simulink model "sim_tcyb_2024_pos_ctrl"  (R2020a)
settings: Solver=ode4  StartTime=0.0  StopTime=30.0  FixedStep=0.01  RelTol=1e-3
values from neighbouring files (symbols this model uses):
  alfa_theta = 20    [init_tcyb_2024_pos_ctrl.m]
  alfa_theta_obs = 100    [init_tcyb_2024_pos_ctrl.m]
  c1_diff_sigma_bar_v = diag([25; 30; 20])    [init_tcyb_2024_pos_ctrl.m]
  c1v = diag([5.8; 6.5; 6.5])    [init_tcyb_2024_pos_ctrl.m]
  c2_diff_sigma_bar_v = diag([50; 50; 10])    [init_tcyb_2024_pos_ctrl.m]
  c2v = diag([5.8; 6.5; 6.5])    [init_tcyb_2024_pos_ctrl.m]
  c3_diff_sigma_bar_v = diag([15; 15; 10])    [init_tcyb_2024_pos_ctrl.m]
  c3v = diag([4.8; 6.4; 6.0])    [init_tcyb_2024_pos_ctrl.m]
  c_psi_p = [0.05; 0.05; 0.05]    [init_tcyb_2024_pos_ctrl.m]
  delta_p_i_0 = zeros(3, NF)    [init_tcyb_2024_pos_ctrl.m]
  delta_v_i_0 = zeros(3, NF)    [init_tcyb_2024_pos_ctrl.m]
  dp_aa_t = 0.2 * ones(3, 5) + ( 1.0 - 0.2 ) * rand(3, 5)    [init_tcyb_2024_pos_ctrl.m]
  dp_ff_t = [ 0.4 * ones(1, 5) + ( 1.0 - 0.4 ) * rand(1, 5);                      0.4 * ones(1, 5) + ( 1.0 - 0.4 ) * rand(1, 5);                      0.2 * ones(1, 5) + ( 0.6 - 0.2 ) * rand(1, 5) ]    [init_tcyb_2024_pos_ctrl.m]
  dp_phi_t = ( - pi / 2 ) * ones(3, 5) + ( pi / 2 - ( - pi / 2 ) ) * rand(3, 5)    [init_tcyb_2024_pos_ctrl.m]
  etai_0 = zeros(3,5)    [init_tcyb_2024_pos_ctrl.m]
  kai_1_t = 0.02    [init_tcyb_2024_pos_ctrl.m]
  kai_3_t = 0.1    [init_tcyb_2024_pos_ctrl.m]
  ksii_0 = zeros(3,5)    [init_tcyb_2024_pos_ctrl.m]
  l1v = diag([20; 20; 20])    [init_tcyb_2024_pos_ctrl.m]
  l2v = diag([30; 30; 30])    [init_tcyb_2024_pos_ctrl.m]
  Lamd_diff_sigma_bar_v = 0.5    [init_tcyb_2024_pos_ctrl.m]
  mass_i = zeros(1,NF)    [init_tcyb_2024_pos_ctrl.m]
  Mii = diag([1;0;0;0;1])    [init_tcyb_2024_pos_ctrl.m]
  pos0 = zeros(3, 1)    [init_tcyb_2024_pos_ctrl.m]
  PZ0 = P0(3)    [init_tcyb_2024_pos_ctrl.m]
  PZ1 = 10    [init_tcyb_2024_pos_ctrl.m]
  Qci_init = repmat([1;0;0;0],1,NF)    [init_tcyb_2024_pos_ctrl.m]
  R0 = 4    [init_tcyb_2024_pos_ctrl.m]
  R1 = 8    [init_tcyb_2024_pos_ctrl.m]
  rho_p = [0.1; 0.1; 0.1]    [init_tcyb_2024_pos_ctrl.m]
  Rx2 = 10    [init_tcyb_2024_pos_ctrl.m]
  Ry2 = 6    [init_tcyb_2024_pos_ctrl.m]
  Rz2 = 4    [init_tcyb_2024_pos_ctrl.m]
  T0 = 0    [init_tcyb_2024_pos_ctrl.m]
  T1 = tseq1    (= 10)    [init_tcyb_2024_pos_ctrl.m]
  T12 = tseq1 + tseq12    (= 20)    [init_tcyb_2024_pos_ctrl.m]
  T2 = tseq1 + tseq12 + tseq2    (= 30)    [init_tcyb_2024_pos_ctrl.m]
  tau_p = 5    [init_tcyb_2024_pos_ctrl.m]
  theta0 = ( 2 / 5 ) * pi    (= 1.25663706144)    [init_tcyb_2024_pos_ctrl.m]
  vel0 = zeros(3, 1)    [init_tcyb_2024_pos_ctrl.m]
  Wij = [0,0,1,0,0;              0,0,1,1,0;              1,0,0,0,1;              0,1,1,0,0;              0,0,1,0,0]    [init_tcyb_2024_pos_ctrl.m]
  X1 = 8    [init_tcyb_2024_pos_ctrl.m]
  X2 = 2    [init_tcyb_2024_pos_ctrl.m]
  X3 = 3    [init_tcyb_2024_pos_ctrl.m]
  Y1 = 10    [init_tcyb_2024_pos_ctrl.m]
  Y2 = 2    [init_tcyb_2024_pos_ctrl.m]
  Y3 = 4    [init_tcyb_2024_pos_ctrl.m]
  Z1 = 4    [init_tcyb_2024_pos_ctrl.m]
  Z2 = -6    [init_tcyb_2024_pos_ctrl.m]
  Z3 = 2    [init_tcyb_2024_pos_ctrl.m]
  zeta_diff_sigma_bar_v = 0.08    [init_tcyb_2024_pos_ctrl.m]
undefined symbols (not defined in the file or in its folder): cal_frac_squ, p_alfav1, p_alfav2, p_gamma1_pos, p_gamma1_vel, p_gamma2_pos, p_gamma2_vel, q_alfav1, q_alfav2, q_gamma1_pos, q_gamma1_vel, q_gamma2_pos, q_gamma2_vel
(part 4 of 4)

== matlab function sim_tcyb_2024_pos_ctrl/trans to column51 ==
  data: x input; y output
function y = fcn(x)
y = x(:);

== matlab function sim_tcyb_2024_pos_ctrl/eta_p_hat adaptive law agent 4 ==
  data: tau_p input; tsim input; d_eta_p_hat_4 output; err_lump_vec input; eta_p_hat_vec input
function d_eta_p_hat_4 = fcn(tau_p, tsim, err_lump_vec, eta_p_hat_vec)
%%%% 计算自适应律
iiuav = 4;
d_eta_p_hat_4 = tau_p * norm(err_lump_vec(:,iiuav), 2) ...
                                - ( 0.1 * exp(-tsim) ) * tau_p .* eta_p_hat_vec(iiuav);

== matlab function sim_tcyb_2024_pos_ctrl/trans to column52 ==
  data: x input; y output
function y = fcn(x)
y = x(:);

== matlab function sim_tcyb_2024_pos_ctrl/trans to column53 ==
  data: x input; y output
function y = fcn(x)
y = x(:);

== matlab function sim_tcyb_2024_pos_ctrl/trans to column54 ==
  data: x input; y output
function y = fcn(x)
y = x(:);

== matlab function sim_tcyb_2024_pos_ctrl/trans to column55 ==
  data: x input; y output
function y = fcn(x)
y = x(:);

== matlab function sim_tcyb_2024_pos_ctrl/trans to column56 ==
  data: x input; y output
function y = fcn(x)
y = x(:);

== matlab function sim_tcyb_2024_pos_ctrl/trans to column57 ==
  data: x input; y output
function y = fcn(x)
y = x(:);

== matlab function sim_tcyb_2024_pos_ctrl/trans to column58 ==
  data: x input; y output
function y = fcn(x)
y = x(:);

== matlab function sim_tcyb_2024_pos_ctrl/trans to column59 ==
  data: x input; y output
function y = fcn(x)
y = x(:);

== matlab function sim_tcyb_2024_pos_ctrl/trans to column60 ==
  data: x input; y output
function y = fcn(x)
y = x(:);

== matlab function sim_tcyb_2024_pos_ctrl/eta_p_hat adaptive law agent 5 ==
  data: tau_p input; tsim input; d_eta_p_hat_5 output; err_lump_vec input; eta_p_hat_vec input
function d_eta_p_hat_5 = fcn(tau_p, tsim, err_lump_vec, eta_p_hat_vec)
%%%% 计算自适应律
iiuav = 5;
d_eta_p_hat_5 = tau_p * norm(err_lump_vec(:,iiuav), 2) ...
                                - ( 0.1 * exp(-tsim) ) * tau_p .* eta_p_hat_vec(iiuav);

== matlab function sim_tcyb_2024_pos_ctrl/combine eta_p_hat adaptive ==
  data: eta_p_hat_1 input; eta_p_hat_vec output; eta_p_hat_2 input; eta_p_hat_3 input; eta_p_hat_4 input; eta_p_hat_5 input
function eta_p_hat_vec = fcn(eta_p_hat_1, eta_p_hat_2, eta_p_hat_3, eta_p_hat_4, eta_p_hat_5)
%%%% 合并领导者位置观测器输出结果
eta_p_hat_vec = [eta_p_hat_1, eta_p_hat_2, eta_p_hat_3, eta_p_hat_4, eta_p_hat_5];

== matlab function sim_tcyb_2024_pos_ctrl/cal auxiliary error Gi agent 1 ==
  data: tsim input; Gi_1 output; err_lump_vec input; eta_p_hat_vec input
function Gi_1 = fcn(tsim, err_lump_vec, eta_p_hat_vec)
%%%% 计算自适应律
iiuav = 1;
Gi_1 = ( ( eta_p_hat_vec(iiuav) ^ 2 ) / ...
                ( norm(err_lump_vec(:,iiuav), 2) * eta_p_hat_vec(iiuav) + 0.1 * exp(-tsim) ) ) ...
                * err_lump_vec(:,iiuav);

== matlab function sim_tcyb_2024_pos_ctrl/cal position and velocity signal tracking errors ==
  data: ksi_i_vec input; err_ksi_vec output; ksi_d_est_vec input; eta_i_vec input; eta_d_est_vec input; err_eta_vec output
function [err_ksi_vec, err_eta_vec] = fcn(ksi_i_vec, ksi_d_est_vec, eta_i_vec, eta_d_est_vec)
%%%% 计算编队跟踪误差
err_ksi_vec = zeros(3,5);
err_eta_vec = zeros(3,5);
for iiuav = 1:5
    err_ksi_vec(:,iiuav) = ksi_i_vec(:,iiuav) - ksi_d_est_vec(:,iiuav);
    err_eta_vec(:,iiuav) = eta_i_vec(:,iiuav) - eta_d_est_vec(:,iiuav);
end

== matlab function sim_tcyb_2024_pos_ctrl/cal auxiliary error Gi agent 2 ==
  data: tsim input; Gi_2 output; err_lump_vec input; eta_p_hat_vec input
function Gi_2 = fcn(tsim, err_lump_vec, eta_p_hat_vec)
%%%% 计算自适应律
iiuav = 2;
Gi_2 = ( ( eta_p_hat_vec(iiuav) ^ 2 ) / ...
                ( norm(err_lump_vec(:,iiuav), 2) * eta_p_hat_vec(iiuav) + 0.1 * exp(-tsim) ) ) ...
                * err_lump_vec(:,iiuav);

== matlab function sim_tcyb_2024_pos_ctrl/cal auxiliary error Gi agent 3 ==
  data: tsim input; Gi_3 output; err_lump_vec input; eta_p_hat_vec input
function Gi_3 = fcn(tsim, err_lump_vec, eta_p_hat_vec)
%%%% 计算自适应律
iiuav = 3;
Gi_3 = ( ( eta_p_hat_vec(iiuav) ^ 2 ) / ...
                ( norm(err_lump_vec(:,iiuav), 2) * eta_p_hat_vec(iiuav) + 0.1 * exp(-tsim) ) ) ...
                * err_lump_vec(:,iiuav);

== matlab function sim_tcyb_2024_pos_ctrl/cal auxiliary error Gi agent 4 ==
  data: tsim input; Gi_4 output; err_lump_vec input; eta_p_hat_vec input
function Gi_4 = fcn(tsim, err_lump_vec, eta_p_hat_vec)
%%%% 计算自适应律
iiuav = 4;
Gi_4 = ( ( eta_p_hat_vec(iiuav) ^ 2 ) / ...
                ( norm(err_lump_vec(:,iiuav), 2) * eta_p_hat_vec(iiuav) + 0.1 * exp(-tsim) ) ) ...
                * err_lump_vec(:,iiuav);

== matlab function sim_tcyb_2024_pos_ctrl/cal auxiliary error Gi agent 5 ==
  data: tsim input; Gi_5 output; err_lump_vec input; eta_p_hat_vec input
function Gi_5 = fcn(tsim, err_lump_vec, eta_p_hat_vec)
%%%% 计算自适应律
iiuav = 5;
Gi_5 = ( ( eta_p_hat_vec(iiuav) ^ 2 ) / ...
                ( norm(err_lump_vec(:,iiuav), 2) * eta_p_hat_vec(iiuav) + 0.1 * exp(-tsim) ) ) ...
                * err_lump_vec(:,iiuav);

== matlab function sim_tcyb_2024_pos_ctrl/combine Gi ==
  data: Gi_1 input; Gi_vec output; Gi_2 input; Gi_3 input; Gi_4 input; Gi_5 input
function Gi_vec = fcn(Gi_1, Gi_2, Gi_3, Gi_4, Gi_5)
%%%% 合并领导者位置观测器输出结果
Gi_vec = [Gi_1(:), Gi_2(:), Gi_3(:), Gi_4(:), Gi_5(:)];

== matlab function sim_tcyb_2024_pos_ctrl/cal formation tracking Gi error ==
  data: wi0 input; err_Gi_form_vec output; wij input; Gi_vec input
function err_Gi_form_vec = fcn(wi0, wij, Gi_vec)
%%%% 计算编队跟踪误差
err_Gi_form_vec = zeros(3,5);
for iiuav = 1:5
    err_Gi_form_vec(:,iiuav) = wi0(iiuav, iiuav) * Gi_vec(:,iiuav);
    for jjuav = 1:5
        err_Gi_form_vec(:,iiuav) = err_Gi_form_vec(:,iiuav) ...
                                                        + wij(iiuav, jjuav) * (Gi_vec(:,iiuav) - Gi_vec(:,jjuav));
    end
end

== matlab function sim_tcyb_2024_pos_ctrl/cal ui agent 2 ==
  data: c_psi_p input; d_delta_eta_vec input; ui_2 output; err_Gi_form_vec input; eps_p_hat_vec input; err_lump_vec input; dp_hat_vec input
function ui_2 = fcn(c_psi_p, d_delta_eta_vec, err_Gi_form_vec, eps_p_hat_vec, err_lump_vec, dp_hat_vec)
%%%% 计算控制输入ui
iiuav = 2;
g0 = 9.80663;
e3 = [0;0;1];
ui_2 = g0 * e3 + d_delta_eta_vec(:,iiuav) - c_psi_p(:) .* err_Gi_form_vec(:,iiuav) ...
            - eps_p_hat_vec(iiuav) * err_lump_vec(:,iiuav) - dp_hat_vec(:,iiuav);

== matlab function sim_tcyb_2024_pos_ctrl/cal ui agent 3 ==
  data: c_psi_p input; d_delta_eta_vec input; ui_3 output; err_Gi_form_vec input; eps_p_hat_vec input; err_lump_vec input; dp_hat_vec input
function ui_3 = fcn(c_psi_p, d_delta_eta_vec, err_Gi_form_vec, eps_p_hat_vec, err_lump_vec, dp_hat_vec)
%%%% 计算控制输入ui
iiuav = 3;
g0 = 9.80663;
e3 = [0;0;1];
ui_3 = g0 * e3 + d_delta_eta_vec(:,iiuav) - c_psi_p(:) .* err_Gi_form_vec(:,iiuav) ...
            - eps_p_hat_vec(iiuav) * err_lump_vec(:,iiuav) - dp_hat_vec(:,iiuav);

== matlab function sim_tcyb_2024_pos_ctrl/cal ui agent 4 ==
  data: c_psi_p input; d_delta_eta_vec input; ui_4 output; err_Gi_form_vec input; eps_p_hat_vec input; err_lump_vec input; dp_hat_vec input
function ui_4 = fcn(c_psi_p, d_delta_eta_vec, err_Gi_form_vec, eps_p_hat_vec, err_lump_vec, dp_hat_vec)
%%%% 计算控制输入ui
iiuav = 4;
g0 = 9.80663;
e3 = [0;0;1];
ui_4 = g0 * e3 + d_delta_eta_vec(:,iiuav) - c_psi_p(:) .* err_Gi_form_vec(:,iiuav) ...
            - eps_p_hat_vec(iiuav) * err_lump_vec(:,iiuav) - dp_hat_vec(:,iiuav);

== matlab function sim_tcyb_2024_pos_ctrl/cal ui agent 5 ==
  data: c_psi_p input; d_delta_eta_vec input; ui_5 output; err_Gi_form_vec input; eps_p_hat_vec input; err_lump_vec input; dp_hat_vec input
function ui_5 = fcn(c_psi_p, d_delta_eta_vec, err_Gi_form_vec, eps_p_hat_vec, err_lump_vec, dp_hat_vec)
%%%% 计算控制输入ui
iiuav = 5;
g0 = 9.80663;
e3 = [0;0;1];
ui_5 = g0 * e3 + d_delta_eta_vec(:,iiuav) - c_psi_p(:) .* err_Gi_form_vec(:,iiuav) ...
            - eps_p_hat_vec(iiuav) * err_lump_vec(:,iiuav) - dp_hat_vec(:,iiuav);

== matlab function sim_tcyb_2024_pos_ctrl/leader control input ==
  data: t input; u0 output; T1 input; T2 input; R0 input; R1 input; Rx2 input; Ry2 input; Rz2 input
function u0  = fcn(t, T1, T2, R0, R1, Rx2, Ry2, Rz2)
%%%% 给出领导者参考加速度控制输入
u0 = zeros(3, 1);

if t <= ( T1 + 1e-05 )
    u0(1, 1) = - ( 4 * pi * sin( ( 2 * pi * ( t - 0 ) ) / ( 0 - T1 ) ) * ( R0 - R1 ) ) / ( ( 0 - T1 ) ^ 2 ) ...
                        - ( 4 * ( pi ^ 2 ) * cos( ( 2 * pi * ( t - 0 ) ) / ( 0 - T1 ) ) ...
                        * ( R0 + ( ( R0 - R1 ) * ( t - 0 ) ) / ( 0 - T1 ) ) ) / ( ( 0 - T1 ) ^ 2 );
    u0(2, 1) = ( 4 * pi * cos( ( 2 * pi * ( t - 0 ) ) / ( 0 - T1 ) ) * ( R0 - R1 ) ) / ( ( 0 - T1 ) ^ 2 ) ...
                        - ( 4 * ( pi ^ 2 ) * sin( ( 2 * pi * ( t - 0 ) ) / ( 0 - T1 ) ) ...
                        * ( R0 + ( ( R0 - R1 ) * ( t - 0 ) ) / ( 0 - T1 ) ) ) / ( ( 0 - T1 ) ^ 2 );
    u0(3, 1) = 0;
else
    u0(1, 1) = ( 4 * Rx2 * ( pi ^ 2 ) * cos( ( 2 * pi * ( t - T1 ) ) / ( T1 - T2 ) ) ) / ( ( T1 - T2 ) ^ 2 );
    u0(2, 1) = - ( 16 * Ry2 * ( pi ^ 2 ) * sin( ( 4 * pi * ( t - T1 ) ) / ( T1 - T2 ) ) ) / ( ( T1 - T2 ) ^ 2 );
    u0(3, 1) = ( 16 * Rz2 * ( pi ^ 2 ) * sin( ( 4 * pi * ( t - T1 ) ) / ( T1 - T2 ) ) ) / ( ( T1 - T2 ) ^ 2 );
end

== matlab function sim_tcyb_2024_pos_ctrl/combine formation control input ==
  data: eta_i_vec output; ksi_i_vec output; eta_1 input; eta_2 input; eta_3 input; eta_4 input; eta_5 input; ksi_1 input; ksi_2 input; ksi_3 input; ksi_4 input; ksi_5 input
function [eta_i_vec, ksi_i_vec] = fcn(eta_1, eta_2, eta_3, eta_4, eta_5, ...
                                                                ksi_1, ksi_2, ksi_3, ksi_4, ksi_5)
%%%% 合并领导者编队跟踪误差结果
eta_i_vec = [eta_1(:), eta_2(:), eta_3(:), eta_4(:), eta_5(:)];
ksi_i_vec = [ksi_1(:), ksi_2(:), ksi_3(:), ksi_4(:), ksi_5(:)];

== matlab function sim_tcyb_2024_pos_ctrl/process velocity ==
  data: T0 input; T1 input; T2 input; PZ0 input; PZ1 input; R0 input; R1 input; Rx2 input; Ry2 input; Rz2 input; t input; V_init_out output
function V_init_out = fcn(T0, T1, T2, PZ0, PZ1, R0, R1, Rx2, Ry2, Rz2, t)
V_init_out = zeros(3, 1);
if t < T1 + 1e-05
    V_init_out(1, 1) = ( cos( ( 2 * pi * ( t - T0 ) ) / ( T0 - T1 ) ) * ( R0 - R1 ) ) / ( T0 - T1 ) ...
                                    - ( 2 * pi * sin( ( 2 * pi * ( t - T0 ) ) / ( T0 - T1 ) ) * ( R0 + ( ( R0 - R1 ) * ( t - T0 ) ) / ( T0 - T1 ) ) ) / ( T0 - T1 );
    V_init_out(2, 1) = ( sin( ( 2 * pi * ( t - T0 ) ) / ( T0 - T1 ) ) * ( R0 - R1 ) ) / ( T0 - T1 ) ...
                                    + ( 2 * pi * cos( ( 2 * pi * ( t - T0 ) ) / ( T0 - T1 ) ) * ( R0 + ( ( R0 - R1 ) * ( t - T0 ) ) / ( T0 - T1 ) ) ) / ( T0 - T1 );
    V_init_out(3, 1) = ( PZ0 - PZ1 ) / ( T0 - T1 );
else
    V_init_out(1, 1) = ( 2 * Rx2 * pi * sin( ( 2 * pi * ( t - T1 ) ) / ( T1 - T2 ) ) ) / ( T1 - T2 );
    V_init_out(2, 1) = ( 4 * Ry2 * pi * cos( ( 4 * pi * ( t - T1 ) ) / ( T1 - T2 ) ) ) / ( T1 - T2 );
    V_init_out(3, 1) = - ( 4 * Rz2 * pi * cos( ( 4 * pi * ( t - T1 ) ) / ( T1 - T2 ) ) ) / ( T1 - T2 );
end

== matlab function sim_tcyb_2024_pos_ctrl/set desire formation configuration ==
  data: X1 input; X2 input; X3 input; Y1 input; Y2 input; Y3 input; Z1 input; Z2 input; Z3 input; theta0 input; kai_1_t input; kai_3_t input; T1 input; T12 input; t input; delta_ksi_vec output; delta_eta_vec output; d_delta_eta_vec output
function [delta_ksi_vec, delta_eta_vec, d_delta_eta_vec] = fcn(X1, X2, X3, Y1, Y2, Y3, Z1, Z2, Z3, ...
                                                                                                                theta0, kai_1_t, kai_3_t, T1, T12, t)
%%%% 计算跟随者期望速度分布式观测器误差
delta_ksi_vec = zeros(3, 5);
delta_eta_vec = zeros(3, 5);
d_delta_eta_vec = zeros(3, 5);
if t <= ( T1 + 1e-04 )
    exp_tmp = exp( -kai_1_t * t );
    delta_ksi_vec(:, 1) = [ X1 * cos( theta0 ) - X2 * exp_tmp; ...
                                            Y1 * sin( theta0 ) - Y2 * exp_tmp; ...
                                            Z1 - Z2 * exp_tmp ];
    delta_ksi_vec(:, 2) = [ - X1 * cos( theta0 ) + X2 * exp_tmp; ...
                                            Y1 * sin( theta0 ) - Y2 * exp_tmp; ...
                                            Z1 + Z2 * exp_tmp ];
    delta_ksi_vec(:, 3) = [ X1 - X2 * exp_tmp; ...
                                            Y2 * exp_tmp; ...
                                            ( 3 / 8 ) * Z1 + Z2 * exp_tmp ];
    delta_ksi_vec(:, 4) = [ - X1 * cos( theta0 ) + X2 * exp_tmp; ...
                                            - Y1 * sin( theta0 ) + Y2 * exp_tmp; ...
                                            Z1 + Z2 * exp_tmp ];
    delta_ksi_vec(:, 5) = [ X1 * cos( theta0 ) - X2 * exp_tmp; ...
                                            - Y1 * sin( theta0 ) + Y2 * exp_tmp; ...
                                            Z1 - Z2 * exp_tmp ];
    delta_eta_vec(:, 1) = [ kai_1_t * X2 * exp_tmp; kai_1_t * Y2 * exp_tmp; kai_1_t * Z2 * exp_tmp ];
    delta_eta_vec(:, 2) = [ - kai_1_t * X2 * exp_tmp; kai_1_t * Y2 * exp_tmp; - kai_1_t * Z2 * exp_tmp ];
    delta_eta_vec(:, 3) = [ kai_1_t * X2 * exp_tmp; - kai_1_t * Y2 * exp_tmp; - kai_1_t * Z2 * exp_tmp ];
    delta_eta_vec(:, 4) = [ - kai_1_t * X2 * exp_tmp; - kai_1_t * Y2 * exp_tmp; - kai_1_t * Z2 * exp_tmp ];
    delta_eta_vec(:, 5) = [ kai_1_t * X2 * exp_tmp; - kai_1_t * Y2 * exp_tmp; kai_1_t * Z2 * exp_tmp ];
    d_delta_eta_vec(:, 1) = [ - ( kai_1_t ^ 2 ) * X2 * exp_tmp; - ( kai_1_t ^ 2 ) * Y2 * exp_tmp; - ( kai_1_t ^ 2 ) * Z2 * exp_tmp ];
    d_delta_eta_vec(:, 2) = [ ( kai_1_t ^ 2 ) * X2 * exp_tmp; - ( kai_1_t ^ 2 ) * Y2 * exp_tmp; ( kai_1_t ^ 2 ) * Z2 * exp_tmp ];
    d_delta_eta_vec(:, 3) = [ - ( kai_1_t ^ 2 ) * X2 * exp_tmp; ( kai_1_t ^ 2 ) * Y2 * exp_tmp; ( kai_1_t ^ 2 ) * Z2 * exp_tmp ];
    d_delta_eta_vec(:, 4) = [ ( kai_1_t ^ 2 ) * X2 * exp_tmp; ( kai_1_t ^ 2 ) * Y2 * exp_tmp; ( kai_1_t ^ 2 ) * Z2 * exp_tmp ];
    d_delta_eta_vec(:, 5) = [ - ( kai_1_t ^ 2 ) * X2 * exp_tmp; ( kai_1_t ^ 2 ) * Y2 * exp_tmp; - ( kai_1_t ^ 2 ) * Z2 * exp_tmp ];
elseif t <= ( T12 + 1e-04 )
    delta_ksi_vec(:, 1) = [ X1 * cos( theta0 ) - X2; Y1 * sin( theta0 ) - Y2; Z1 - Z2 ];
    delta_ksi_vec(:, 2) = [ - X1 * cos( theta0 ) + X2; Y1 * sin( theta0 ) - Y2; Z1 + Z2 ];
    delta_ksi_vec(:, 3) = [ X1 - X2; 0; ( 3 / 8 ) * Z1 + Z2 ];
    delta_ksi_vec(:, 4) = [ - X1 * cos( theta0 ) + X2; - Y1 * sin( theta0 ) + Y2; Z1 + Z2 ];
    delta_ksi_vec(:, 5) = [ X1 * cos( theta0 ) - X2; - Y1 * sin( theta0 ) + Y2; Z1 - Z2 ];
else
    exp_tmp = 1 / ( 1 + exp( - kai_3_t * ( t - T12 - 5 ) ) );
    tmp_2 = exp( - kai_3_t * ( t - T12 - 5 ) ) / ( ( 1 + exp( - kai_3_t * ( t - T12 - 5 ) ) ) ^ 2 );
    delta_ksi_vec(:, 1) = [ X1 * cos( theta0 ) - X2 + X3 * exp_tmp; ...
                                            Y1 * sin( theta0 ) - Y2 + Y3 * exp_tmp; ...
                                            Z1 - Z2 + Z3 * exp_tmp ];
    delta_ksi_vec(:, 2) = [ - X1 * cos( theta0 ) + X2 - X3 * exp_tmp; ...
                                            Y1 * sin( theta0 ) - Y2 + Y3 * exp_tmp; ...
                                            Z1 + Z2 - Z3 * exp_tmp ];
    delta_ksi_vec(:, 3) = [ X1 - X2 + X3 * exp_tmp; ...
                                            - Y3 * exp_tmp; ...
                                            ( 3 / 8 ) * Z1 + Z2 - Z3 * exp_tmp ];
    delta_ksi_vec(:, 4) = [ - X1 * cos( theta0 ) + X2 - X3 * exp_tmp; ...
                                            - Y1 * sin( theta0 ) + Y2 - Y3 * exp_tmp; ...
                                            Z1 + Z2 - Z3 * exp_tmp ];
    delta_ksi_vec(:, 5) = [ X1 * cos( theta0 ) - X2 + X3 * exp_tmp; ...
                                            - Y1 * sin( theta0 ) + Y2 - Y3 * exp_tmp; ...
                                            Z1 - Z2 + Z3 * exp_tmp ];
    delta_eta_vec(:, 1) = [ kai_3_t * X3 * tmp_2; kai_3_t * Y3 * tmp_2; kai_3_t * Z3 * tmp_2 ];
    delta_eta_vec(:, 2) = [ - kai_3_t * X3 * tmp_2; kai_3_t * Y3 * tmp_2; kai_3_t * Z3 * tmp_2 ];
    delta_eta_vec(:, 3) = [ kai_3_t * X3 * tmp_2; - kai_3_t * Y3 * tmp_2; - kai_3_t * Z3 * tmp_2 ];
    delta_eta_vec(:, 4) = [ - kai_3_t * X3 * tmp_2; - kai_3_t * Y3 * tmp_2; - kai_3_t * Z3 * tmp_2 ];
    delta_eta_vec(:, 5) = [ kai_3_t * X3 * tmp_2; kai_3_t * Y3 * tmp_2; - kai_3_t * Z3 * tmp_2 ];
    d_delta_eta_vec(:, 1) = ( kai_3_t * ( 1 - exp( - kai_3_t * ( t - T12 - 5 ) ) ) * exp_tmp ) * delta_eta_vec(:, 1);
    d_delta_eta_vec(:, 2) = ( kai_3_t * ( 1 - exp( - kai_3_t * ( t - T12 - 5 ) ) ) * exp_tmp ) * delta_eta_vec(:, 2);
    d_delta_eta_vec(:, 3) = ( kai_3_t * ( 1 - exp( - kai_3_t * ( t - T12 - 5 ) ) ) * exp_tmp ) * delta_eta_vec(:, 3);
    d_delta_eta_vec(:, 4) = ( kai_3_t * ( 1 - exp( - kai_3_t * ( t - T12 - 5 ) ) ) * exp_tmp ) * delta_eta_vec(:, 4);
    d_delta_eta_vec(:, 5) = ( kai_3_t * ( 1 - exp( - kai_3_t * ( t - T12 - 5 ) ) ) * exp_tmp ) * delta_eta_vec(:, 5);
end

== matlab function sim_tcyb_2024_pos_ctrl/uav translational dynamics agent 1 ==
  data: dvi output; Ri input; ui input; dp input
function dvi = fcn(Ri, ui, dp)
%%%% 根据控制输入计算无人机平移动力学微分方程
iiuav = 1;
g0 = 9.80663;
e3 = [0;0;1];
dvi = -g0 * e3 + norm(ui(:,iiuav),2) * Ri(:,:,iiuav) * e3 + dp(:,iiuav);

== matlab function sim_tcyb_2024_pos_ctrl/uav translational dynamics agent 2 ==
  data: dvi output; Ri input; ui input; dp input
function dvi = fcn(Ri, ui, dp)
%%%% 根据控制输入计算无人机平移动力学微分方程
iiuav = 2;
g0 = 9.80663;
e3 = [0;0;1];
dvi = -g0 * e3 + norm(ui(:,iiuav),2) * Ri(:,:,iiuav) * e3 + dp(:,iiuav);

== matlab function sim_tcyb_2024_pos_ctrl/uav translational dynamics agent 3 ==
  data: dvi output; Ri input; ui input; dp input
function dvi = fcn(Ri, ui, dp)
%%%% 根据控制输入计算无人机平移动力学微分方程
iiuav = 3;
g0 = 9.80663;
e3 = [0;0;1];
dvi = -g0 * e3 + norm(ui(:,iiuav),2) * Ri(:,:,iiuav) * e3 + dp(:,iiuav);

== matlab function sim_tcyb_2024_pos_ctrl/uav translational dynamics agent 4 ==
  data: dvi output; Ri input; ui input; dp input
function dvi = fcn(Ri, ui, dp)
%%%% 根据控制输入计算无人机平移动力学微分方程
iiuav = 4;
g0 = 9.80663;
e3 = [0;0;1];
dvi = -g0 * e3 + norm(ui(:,iiuav),2) * Ri(:,:,iiuav) * e3 + dp(:,iiuav);

== matlab function sim_tcyb_2024_pos_ctrl/uav translational dynamics agent 5 ==
  data: dvi output; Ri input; ui input; dp input
function dvi = fcn(Ri, ui, dp)
%%%% 根据控制输入计算无人机平移动力学微分方程
iiuav = 5;
g0 = 9.80663;
e3 = [0;0;1];
dvi = -g0 * e3 + norm(ui(:,iiuav),2) * Ri(:,:,iiuav) * e3 + dp(:,iiuav);

== matlab function sim_tcyb_2024_pos_ctrl/cal Ri ==
  data: Ri output; Rei input; Rci input
function Ri = fcn(Rei, Rci)
%%%% 使用罗德里格公式由四元数Qci求解Rci
Ri = zeros(3,3,5);
for iiuav = 1:5
    Ri(:,:,iiuav) = Rci(:,:,iiuav) * Rei(:,:,iiuav);
end

end

== matlab function sim_tcyb_2024_pos_ctrl/follower tracking error agent 1 ==
  data: ksi_track_err_1 output; delta_ksi_vec input; delta_eta_vec input; ksi_i_vec input; eta_i_vec input; ksi0 input; eta_track_err_1 output; eta0 input
function [ksi_track_err_1, eta_track_err_1]  = fcn(delta_ksi_vec, delta_eta_vec, ksi_i_vec, eta_i_vec, ksi0, eta0)
%%%% 计算跟随者节点1号位置/速度跟踪误差
eta_track_err_1 = eta_i_vec(:,1) - delta_eta_vec(:,1) - eta0;
ksi_track_err_1 = ksi_i_vec(:,1) - delta_ksi_vec(:,1) - ksi0;

== matlab function sim_tcyb_2024_pos_ctrl/follower tracking error agent 2 ==
  data: ksi_track_err_2 output; delta_ksi_vec input; delta_eta_vec input; ksi_i_vec input; eta_i_vec input; ksi0 input; eta_track_err_2 output; eta0 input
function [ksi_track_err_2, eta_track_err_2]  = fcn(delta_ksi_vec, delta_eta_vec, ksi_i_vec, eta_i_vec, ksi0, eta0)
%%%% 计算跟随者节点2号位置/速度跟踪误差
eta_track_err_2 = eta_i_vec(:,2) - delta_eta_vec(:,2) - eta0;
ksi_track_err_2 = ksi_i_vec(:,2) - delta_ksi_vec(:,2) - ksi0;

== matlab function sim_tcyb_2024_pos_ctrl/follower tracking error agent 3 ==
  data: ksi_track_err_3 output; delta_ksi_vec input; delta_eta_vec input; ksi_i_vec input; eta_i_vec input; ksi0 input; eta_track_err_3 output; eta0 input
function [ksi_track_err_3, eta_track_err_3]  = fcn(delta_ksi_vec, delta_eta_vec, ksi_i_vec, eta_i_vec, ksi0, eta0)
%%%% 计算跟随者节点3号位置/速度跟踪误差
eta_track_err_3 = eta_i_vec(:,3) - delta_eta_vec(:,3) - eta0;
ksi_track_err_3 = ksi_i_vec(:,3) - delta_ksi_vec(:,3) - ksi0;

== matlab function sim_tcyb_2024_pos_ctrl/follower tracking error agent 4 ==
  data: ksi_track_err_4 output; delta_ksi_vec input; delta_eta_vec input; ksi_i_vec input; eta_i_vec input; ksi0 input; eta_track_err_4 output; eta0 input
function [ksi_track_err_4, eta_track_err_4]  = fcn(delta_ksi_vec, delta_eta_vec, ksi_i_vec, eta_i_vec, ksi0, eta0)
%%%% 计算跟随者节点4号位置/速度跟踪误差
eta_track_err_4 = eta_i_vec(:,4) - delta_eta_vec(:,4) - eta0;
ksi_track_err_4 = ksi_i_vec(:,4) - delta_ksi_vec(:,4) - ksi0;

== matlab function sim_tcyb_2024_pos_ctrl/follower tracking error agent 5 ==
  data: ksi_track_err_5 output; delta_ksi_vec input; delta_eta_vec input; ksi_i_vec input; eta_i_vec input; ksi0 input; eta_track_err_5 output; eta0 input
function [ksi_track_err_5, eta_track_err_5]  = fcn(delta_ksi_vec, delta_eta_vec, ksi_i_vec, eta_i_vec, ksi0, eta0)
%%%% 计算跟随者节点5号位置/速度跟踪误差
eta_track_err_5 = eta_i_vec(:,5) - delta_eta_vec(:,5) - eta0;
ksi_track_err_5 = ksi_i_vec(:,5) - delta_ksi_vec(:,5) - ksi0;

== matlab function sim_tcyb_2024_pos_ctrl/combine follower eta ksi ==
  data: ksi_track_err_vec output; ksi_track_err_1 input; ksi_track_err_2 input; ksi_track_err_3 input; ksi_track_err_4 input; ksi_track_err_5 input; eta_track_err_vec output; eta_track_err_1 input; eta_track_err_2 input; eta_track_err_3 input; eta_track_err_4 input; eta_track_err_5 input
function [ksi_track_err_vec, eta_track_err_vec]  = fcn(ksi_track_err_1, ksi_track_err_2, ksi_track_err_3, ksi_track_err_4, ksi_track_err_5, ...
                                                                                    eta_track_err_1, eta_track_err_2, eta_track_err_3, eta_track_err_4, eta_track_err_5)
%%%% 合并所有跟随者的速度/位置向量
ksi_track_err_vec = [ksi_track_err_1(:), ksi_track_err_2(:), ksi_track_err_3(:), ksi_track_err_4(:), ksi_track_err_5(:)];
eta_track_err_vec = [eta_track_err_1(:), eta_track_err_2(:), eta_track_err_3(:), eta_track_err_4(:), eta_track_err_5(:)];

== matlab function sim_tcyb_2024_pos_ctrl/depart Rc5 ==
  data: y output; x input
function y = fcn(x)
y = x(:,:,5);

end

== matlab function sim_tcyb_2024_pos_ctrl/depart Rc1 ==
  data: y output; x input
function y = fcn(x)
y = x(:,:,1);

end

== matlab function sim_tcyb_2024_pos_ctrl/depart Rc2 ==
  data: y output; x input
function y = fcn(x)
y = x(:,:,2);

end

== matlab function sim_tcyb_2024_pos_ctrl/depart Rc3 ==
  data: y output; x input
function y = fcn(x)
y = x(:,:,3);

end

== matlab function sim_tcyb_2024_pos_ctrl/depart Rc4 ==
  data: y output; x input
function y = fcn(x)
y = x(:,:,4);

end

== matlab function sim_tcyb_2024_pos_ctrl/cal virtual control sigma_v agent 1 ==
  data: c3v input; Ri input; ui_vec input; d_sigma_v_1 output; sigma_bar_v_vec input
function d_sigma_v_1 = fcn(c3v, Ri, ui_vec, sigma_bar_v_vec)
%%%% 计算扰动观测器中虚拟速度控制量sigma_v的微分方程

iiuav = 1;
g0 = 9.80663;
e3 = [0;0;1];
d_sigma_v_1 = -g0 * e3 + norm(ui_vec(:,iiuav), 2) * Ri(:,:,iiuav) * e3 + c3v * sigma_bar_v_vec(:,iiuav);

== matlab function sim_tcyb_2024_pos_ctrl/cal virtual control sigma_v agent 2 ==
  data: c3v input; Ri input; ui_vec input; d_sigma_v_2 output; sigma_bar_v_vec input
function d_sigma_v_2 = fcn(c3v, Ri, ui_vec, sigma_bar_v_vec)
%%%% 计算扰动观测器中虚拟速度控制量sigma_v的微分方程

iiuav = 2;
g0 = 9.80663;
e3 = [0;0;1];
d_sigma_v_2 = -g0 * e3 + norm(ui_vec(:,iiuav), 2) * Ri(:,:,iiuav) * e3 + c3v * sigma_bar_v_vec(:,iiuav);

== matlab function sim_tcyb_2024_pos_ctrl/cal virtual control sigma_v agent 3 ==
  data: c3v input; Ri input; ui_vec input; d_sigma_v_3 output; sigma_bar_v_vec input
function d_sigma_v_3 = fcn(c3v, Ri, ui_vec, sigma_bar_v_vec)
%%%% 计算扰动观测器中虚拟速度控制量sigma_v的微分方程

iiuav = 3;
g0 = 9.80663;
e3 = [0;0;1];
d_sigma_v_3 = -g0 * e3 + norm(ui_vec(:,iiuav), 2) * Ri(:,:,iiuav) * e3 + c3v * sigma_bar_v_vec(:,iiuav);

== matlab function sim_tcyb_2024_pos_ctrl/cal virtual control sigma_v agent 4 ==
  data: c3v input; Ri input; ui_vec input; d_sigma_v_4 output; sigma_bar_v_vec input
function d_sigma_v_4 = fcn(c3v, Ri, ui_vec, sigma_bar_v_vec)
%%%% 计算扰动观测器中虚拟速度控制量sigma_v的微分方程

iiuav = 4;
g0 = 9.80663;
e3 = [0;0;1];
d_sigma_v_4 = -g0 * e3 + norm(ui_vec(:,iiuav), 2) * Ri(:,:,iiuav) * e3 + c3v * sigma_bar_v_vec(:,iiuav);

== matlab function sim_tcyb_2024_pos_ctrl/cal virtual control sigma_v agent 5 ==
  data: c3v input; Ri input; ui_vec input; d_sigma_v_5 output; sigma_bar_v_vec input
function d_sigma_v_5 = fcn(c3v, Ri, ui_vec, sigma_bar_v_vec)
%%%% 计算扰动观测器中虚拟速度控制量sigma_v的微分方程

iiuav = 5;
g0 = 9.80663;
e3 = [0;0;1];
d_sigma_v_5 = -g0 * e3 + norm(ui_vec(:,iiuav), 2) * Ri(:,:,iiuav) * e3 + c3v * sigma_bar_v_vec(:,iiuav);

== matlab function sim_tcyb_2024_pos_ctrl/combine sigma_v ==
  data: sigma_v_1 input; sigma_v_2 input; sigma_v_3 input; sigma_v_4 input; sigma_v_5 input; sigma_v_vec output
function sigma_v_vec  = fcn(sigma_v_1, sigma_v_2, sigma_v_3, sigma_v_4, sigma_v_5)
%%%% 合并虚拟速度控制量sigma_v
sigma_v_vec = [sigma_v_1(:), sigma_v_2(:), sigma_v_3(:), sigma_v_4(:), sigma_v_5(:)];

== matlab function sim_tcyb_2024_pos_ctrl/cal combine sigma_bar_v ==
  data: eta_i_vec input; sigma_v_vec input; sigma_bar_v_vec output
function sigma_bar_v_vec = fcn(eta_i_vec, sigma_v_vec)
%%%% 计算虚拟速度追踪误差sigma_bar_v
sigma_bar_v_vec = zeros(3,5);
for iiuav = 1:5
    sigma_bar_v_vec(:,iiuav) = eta_i_vec(:,iiuav) - sigma_v_vec(:,iiuav);
end

== matlab function sim_tcyb_2024_pos_ctrl/cal differentiator d_sigma_bar_v_hat agent 1/cal differentiator ==
  data: c1 input; d_sigma_bar_v_hat output; d_dsigma_bar_v_hat output; d_d2sigma_bar_v_hat output; c2 input; c3 input; chi_t input; sigma_bar_v_sig_1 input; sigma_bar_v_sig_2 input; sigma_bar_v_sig_3 input; sigma_bar_v_sig_4 input; sigma_bar_v_sig_5 input; sigma_bar_v_sig_6 input; d_sigma_bar_v_hat input; d2_sigma_bar_v_hat input
function [d_sigma_bar_v_hat, d_dsigma_bar_v_hat, d_d2sigma_bar_v_hat] = fcn(c1, c2, c3, chi_t, sigma_bar_v_sig_1, sigma_bar_v_sig_2, sigma_bar_v_sig_3, ...
                                                                                                                                                sigma_bar_v_sig_4, sigma_bar_v_sig_5, sigma_bar_v_sig_6, d_sigma_bar_v_hat, d2_sigma_bar_v_hat)
d_d2sigma_bar_v_hat = -chi_t .* c1 * sigma_bar_v_sig_1(:) - (1 - chi_t) .* c1 * sigma_bar_v_sig_2(:);
d_dsigma_bar_v_hat = -chi_t .* c2 * sigma_bar_v_sig_3(:) - (1 - chi_t) .* c2 * sigma_bar_v_sig_4(:) + d2_sigma_bar_v_hat(:);
d_sigma_bar_v_hat = -chi_t .* c3 * sigma_bar_v_sig_5(:) - (1 - chi_t) .* c3 * sigma_bar_v_sig_6(:) + d_sigma_bar_v_hat(:);

== matlab function sim_tcyb_2024_pos_ctrl/cal differentiator d_sigma_bar_v_hat agent 1/cal sig ==
  data: x input; z output; y input
function z = fcn(x, y)
z = x(:) .* sign(y(:));

== matlab function sim_tcyb_2024_pos_ctrl/cal differentiator d_sigma_bar_v_hat agent 1/cal sig1 ==
  data: x input; z output; y input
function z = fcn(x, y)
z = x(:) .* sign(y(:));

== matlab function sim_tcyb_2024_pos_ctrl/generate translational disturbance agent 1 ==
  data: dp_aa_t input; dp_ff_t input; dp_phi_t input; dp_1 output; t input
function dp_1 = fcn(dp_aa_t, dp_ff_t, dp_phi_t, t)
%%%% 平移动力学方程中的扰动项设置
epsil_t = zeros(3, 1);

for kk = 1:5
    epsil_t = epsil_t + dp_aa_t(:, kk) .* sin( 2 * pi * dp_ff_t(:, kk) * t + dp_phi_t(:, kk) );
end

dp_1 = [ epsil_t(1) + 1.6 * sin( 0.4 * t ) + 2.0 * cos( 0.5 * t ) + 1.4 * sin( 0.7 * t ) ...
                + 4 * exp( -0.1 * t ) * sin( 0.8 * t ) + 3 / ( 1 + exp( -0.2 * ( t - 15 ) ) ); ...
                epsil_t(2) + 1.2 * sin( 0.2 * t ) + 3 * cos( 0.4 * t ) + 0.8 * sin( 0.6 * t ) ...
                + 2 * exp( -0.15 * t ) * cos( 1.2 * t ) + 3 / ( 1 + exp( -0.3 * ( t - 25 ) ) ); ...
                epsil_t(3) + 1.8 * sin( 0.2 * t ) + 1.6 * sin( 0.3 * t ) + 1.6 * cos( 0.4 * t ) ...
                + 4 * exp( -0.05 * t ) * sin( 0.5 * t + pi / 4 ) + 3 / ( 1 + exp( -0.5 * ( t - 20 ) ) ) ];

== matlab function sim_tcyb_2024_pos_ctrl/cal differentiator d_sigma_bar_v_hat agent 1/cal sig2 ==
  data: x input; z output; y input
function z = fcn(x, y)
z = x(:) .* sign(y(:));

== matlab function sim_tcyb_2024_pos_ctrl/cal differentiator d_sigma_bar_v_hat agent 1/cal sig3 ==
  data: x input; z output; y input
function z = fcn(x, y)
z = x(:) .* sign(y(:));

== matlab function sim_tcyb_2024_pos_ctrl/cal differentiator d_sigma_bar_v_hat agent 1/cal sig4 ==
  data: x input; z output; y input
function z = fcn(x, y)
z = x(:) .* sign(y(:));

== matlab function sim_tcyb_2024_pos_ctrl/cal differentiator d_sigma_bar_v_hat agent 1/cal sig5 ==
  data: x input; z output; y input
function z = fcn(x, y)
z = x(:) .* sign(y(:));

== matlab function sim_tcyb_2024_pos_ctrl/cal differentiator d_sigma_bar_v_hat agent 1/choose sigma_bar_v ==
  data: x input; y output
function y = fcn(x)
iiuav = 1;
y = x(:,iiuav);

== matlab function sim_tcyb_2024_pos_ctrl/cal differentiator d_sigma_bar_v_hat agent 1/trans to column20 ==
  data: x input; y output
function y = fcn(x)
y = x(:);

== matlab function sim_tcyb_2024_pos_ctrl/cal differentiator d_sigma_bar_v_hat agent 1/trans to column21 ==
  data: x input; y output
function y = fcn(x)
y = x(:);

== matlab function sim_tcyb_2024_pos_ctrl/cal differentiator d_sigma_bar_v_hat agent 1/trans to column22 ==
  data: x input; y output
function y = fcn(x)
y = x(:);

== matlab function sim_tcyb_2024_pos_ctrl/cal differentiator d_sigma_bar_v_hat agent 1/trans to column23 ==
  data: x input; y output
function y = fcn(x)
y = x(:);

== matlab function sim_tcyb_2024_pos_ctrl/cal differentiator d_sigma_bar_v_hat agent 1/trans to column24 ==
  data: x input; y output
function y = fcn(x)
y = x(:);

== matlab function sim_tcyb_2024_pos_ctrl/cal differentiator d_sigma_bar_v_hat agent 1/trans to column25 ==
  data: x input; y output
function y = fcn(x)
y = x(:);

== matlab function sim_tcyb_2024_pos_ctrl/cal differentiator d_sigma_bar_v_hat agent 2/cal differentiator ==
  data: c1 input; d_sigma_bar_v_hat output; d_dsigma_bar_v_hat output; d_d2sigma_bar_v_hat output; c2 input; c3 input; chi_t input; sigma_bar_v_sig_1 input; sigma_bar_v_sig_2 input; sigma_bar_v_sig_3 input; sigma_bar_v_sig_4 input; sigma_bar_v_sig_5 input; sigma_bar_v_sig_6 input; d_sigma_bar_v_hat input; d2_sigma_bar_v_hat input
function [d_sigma_bar_v_hat, d_dsigma_bar_v_hat, d_d2sigma_bar_v_hat] = fcn(c1, c2, c3, chi_t, sigma_bar_v_sig_1, sigma_bar_v_sig_2, sigma_bar_v_sig_3, ...
                                                                                                                                                sigma_bar_v_sig_4, sigma_bar_v_sig_5, sigma_bar_v_sig_6, d_sigma_bar_v_hat, d2_sigma_bar_v_hat)
d_d2sigma_bar_v_hat = -chi_t .* c1 * sigma_bar_v_sig_1(:) - (1 - chi_t) .* c1 * sigma_bar_v_sig_2(:);
d_dsigma_bar_v_hat = -chi_t .* c2 * sigma_bar_v_sig_3(:) - (1 - chi_t) .* c2 * sigma_bar_v_sig_4(:) + d2_sigma_bar_v_hat(:);
d_sigma_bar_v_hat = -chi_t .* c3 * sigma_bar_v_sig_5(:) - (1 - chi_t) .* c3 * sigma_bar_v_sig_6(:) + d_sigma_bar_v_hat(:);

== matlab function sim_tcyb_2024_pos_ctrl/generate translational disturbance agent 2 ==
  data: dp_aa_t input; dp_ff_t input; dp_phi_t input; dp_2 output; t input
function dp_2 = fcn(dp_aa_t, dp_ff_t, dp_phi_t, t)
%%%% 平移动力学方程中的扰动项设置
epsil_t = zeros(3, 1);

for kk = 1:5
    epsil_t = epsil_t + dp_aa_t(:, kk) .* sin( 2 * pi * dp_ff_t(:, kk) * t + dp_phi_t(:, kk) );
end

dp_2 = [ epsil_t(1) + 1.6 * sin( 0.2 * t ) + 2.0 * cos( 0.3 * t ) + 1.4 * sin( 0.5 * t ) ...
                + 4 * exp( -0.1 * t ) * sin( 0.5 * t ) + 3 / ( 1 + exp( -0.2 * ( t - 15 ) ) ); ...
                epsil_t(2) + 1.2 * sin( 0.1 * t ) + 3 * cos( 0.2 * t ) + 0.8 * sin( 0.4 * t ) ...
                + 2 * exp( -0.15 * t ) * cos( 0.6 * t ) + 3 / ( 1 + exp( -0.3 * ( t - 25 ) ) ); ...
                epsil_t(3) + 1.8 * sin( 0.1 * t ) + 1.6 * sin( 0.2 * t ) + 1.6 * cos( 0.3 * t ) ...
                + 4 * exp( -0.05 * t ) * sin( 0.4 * t + pi / 4 ) + 3 / ( 1 + exp( -0.5 * ( t - 20 ) ) ) ];

== matlab function sim_tcyb_2024_pos_ctrl/cal Rei ==
  data: Rei output; Qei input
function Rei = fcn(Qei)
%%%% 使用罗德里格公式由四元数Qei求解Rei
Rei = zeros(3,3,5);
for iuav = 1:5
    thetaei_tmp = Qei(1,iuav);
    qei_tmp = Qei(2:4,iuav);
    Rei(:,:,iuav) = ((thetaei_tmp^2) - (qei_tmp')*qei_tmp) * eye(3,3) ...
                            + 2 * qei_tmp * (qei_tmp') ...
                            - 2 * thetaei_tmp * cal_askew_mat(qei_tmp);
end

end

== matlab function sim_tcyb_2024_pos_ctrl/cal differentiator d_sigma_bar_v_hat agent 2/cal sig ==
  data: x input; z output; y input
function z = fcn(x, y)
z = x(:) .* sign(y(:));

== matlab function sim_tcyb_2024_pos_ctrl/cal differentiator d_sigma_bar_v_hat agent 2/cal sig1 ==
  data: x input; z output; y input
function z = fcn(x, y)
z = x(:) .* sign(y(:));

== matlab function sim_tcyb_2024_pos_ctrl/cal differentiator d_sigma_bar_v_hat agent 2/cal sig2 ==
  data: x input; z output; y input
function z = fcn(x, y)
z = x(:) .* sign(y(:));

== matlab function sim_tcyb_2024_pos_ctrl/cal differentiator d_sigma_bar_v_hat agent 2/cal sig3 ==
  data: x input; z output; y input
function z = fcn(x, y)
z = x(:) .* sign(y(:));

== matlab function sim_tcyb_2024_pos_ctrl/cal differentiator d_sigma_bar_v_hat agent 2/cal sig4 ==
  data: x input; z output; y input
function z = fcn(x, y)
z = x(:) .* sign(y(:));

== matlab function sim_tcyb_2024_pos_ctrl/cal differentiator d_sigma_bar_v_hat agent 2/cal sig5 ==
  data: x input; z output; y input
function z = fcn(x, y)
z = x(:) .* sign(y(:));

== matlab function sim_tcyb_2024_pos_ctrl/cal differentiator d_sigma_bar_v_hat agent 2/choose sigma_bar_v ==
  data: x input; y output
function y = fcn(x)
iiuav = 2;
y = x(:,iiuav);

== matlab function sim_tcyb_2024_pos_ctrl/cal differentiator d_sigma_bar_v_hat agent 2/trans to column20 ==
  data: x input; y output
function y = fcn(x)
y = x(:);

== matlab function sim_tcyb_2024_pos_ctrl/cal differentiator d_sigma_bar_v_hat agent 2/trans to column21 ==
  data: x input; y output
function y = fcn(x)
y = x(:);

== matlab function sim_tcyb_2024_pos_ctrl/cal differentiator d_sigma_bar_v_hat agent 2/trans to column22 ==
  data: x input; y output
function y = fcn(x)
y = x(:);

== matlab function sim_tcyb_2024_pos_ctrl/cal differentiator d_sigma_bar_v_hat agent 2/trans to column23 ==
  data: x input; y output
function y = fcn(x)
y = x(:);

== matlab function sim_tcyb_2024_pos_ctrl/cal differentiator d_sigma_bar_v_hat agent 2/trans to column24 ==
  data: x input; y output
function y = fcn(x)
y = x(:);

== matlab function sim_tcyb_2024_pos_ctrl/generate translational disturbance agent 3 ==
  data: dp_aa_t input; dp_ff_t input; dp_phi_t input; dp_3 output; t input
function dp_3 = fcn(dp_aa_t, dp_ff_t, dp_phi_t, t)
%%%% 平移动力学方程中的扰动项设置
epsil_t = zeros(3, 1);

for kk = 1:5
    epsil_t = epsil_t + dp_aa_t(:, kk) .* sin( 2 * pi * dp_ff_t(:, kk) * t + dp_phi_t(:, kk) );
end

dp_3 = [ epsil_t(1) + 1.6 * sin( 0.2 * t ) + 2.0 * cos( 0.3 * t ) + 1.4 * sin( 0.5 * t ) ...
                + 4 * exp( -0.1 * t ) * sin( 0.5 * t ) + 3 / ( 1 + exp( -0.2 * ( t - 15 ) ) ); ...
                epsil_t(2) + 1.2 * sin( 0.1 * t ) + 3 * cos( 0.2 * t ) + 0.8 * sin( 0.4 * t ) ...
                + 2 * exp( -0.15 * t ) * cos( 0.6 * t ) + 3 / ( 1 + exp( -0.3 * ( t - 25 ) ) ); ...
                epsil_t(3) + 1.8 * sin( 0.1 * t ) + 1.6 * sin( 0.2 * t ) + 1.6 * cos( 0.3 * t ) ...
                + 4 * exp( -0.05 * t ) * sin( 0.4 * t + pi / 4 ) + 3 / ( 1 + exp( -0.5 * ( t - 20 ) ) ) ];

== matlab function sim_tcyb_2024_pos_ctrl/cal differentiator d_sigma_bar_v_hat agent 2/trans to column25 ==
  data: x input; y output
function y = fcn(x)
y = x(:);

== matlab function sim_tcyb_2024_pos_ctrl/cal differentiator d_sigma_bar_v_hat agent 3/cal differentiator ==
  data: c1 input; d_sigma_bar_v_hat output; d_dsigma_bar_v_hat output; d_d2sigma_bar_v_hat output; c2 input; c3 input; chi_t input; sigma_bar_v_sig_1 input; sigma_bar_v_sig_2 input; sigma_bar_v_sig_3 input; sigma_bar_v_sig_4 input; sigma_bar_v_sig_5 input; sigma_bar_v_sig_6 input; d_sigma_bar_v_hat input; d2_sigma_bar_v_hat input
function [d_sigma_bar_v_hat, d_dsigma_bar_v_hat, d_d2sigma_bar_v_hat] = fcn(c1, c2, c3, chi_t, sigma_bar_v_sig_1, sigma_bar_v_sig_2, sigma_bar_v_sig_3, ...
                                                                                                                                                sigma_bar_v_sig_4, sigma_bar_v_sig_5, sigma_bar_v_sig_6, d_sigma_bar_v_hat, d2_sigma_bar_v_hat)
d_d2sigma_bar_v_hat = -chi_t .* c1 * sigma_bar_v_sig_1(:) - (1 - chi_t) .* c1 * sigma_bar_v_sig_2(:);
d_dsigma_bar_v_hat = -chi_t .* c2 * sigma_bar_v_sig_3(:) - (1 - chi_t) .* c2 * sigma_bar_v_sig_4(:) + d2_sigma_bar_v_hat(:);
d_sigma_bar_v_hat = -chi_t .* c3 * sigma_bar_v_sig_5(:) - (1 - chi_t) .* c3 * sigma_bar_v_sig_6(:) + d_sigma_bar_v_hat(:);

== matlab function sim_tcyb_2024_pos_ctrl/cal differentiator d_sigma_bar_v_hat agent 3/cal sig ==
  data: x input; z output; y input
function z = fcn(x, y)
z = x(:) .* sign(y(:));

== matlab function sim_tcyb_2024_pos_ctrl/depart Re5 ==
  data: y output; x input
function y = fcn(x)
y = x(:,:,5);

end

== matlab function sim_tcyb_2024_pos_ctrl/depart Re1 ==
  data: y output; x input
function y = fcn(x)
y = x(:,:,1);

end
